simulink model "Assignment1_2"  (R2021a)
settings: Solver=VariableStepAuto  StartTime=0.0  StopTime=10.0  RelTol=1e-3
settings Model: Creator=mstra  LastModifiedBy=Luca
settings SolverCC: AlgebraicLoopSolver=TrustRegion
settings DebuggingCC: SFMachineParentedDataDiag=warning

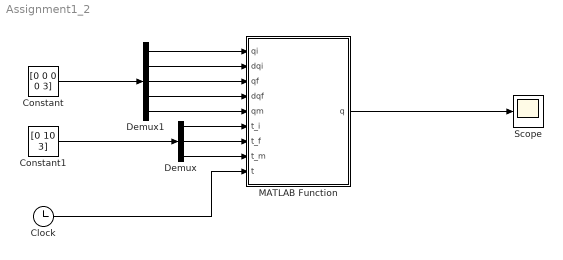
== system Assignment1_2 ==
  Clock : Clock
  Constant : Constant  Value=[0 0 0 0 3]
  Constant1 : Constant  Value=[0 10 3]
  Demux : Demux  Outputs=3
  Demux1 : Demux  Outputs=5
  MATLAB Function : MATLAB Function  TreatAsAtomicUnit=on
  Scope : Scope
  wires:
  Demux/1 -> MATLAB Function/6(t_i)
  Demux/2 -> MATLAB Function/7(t_f)
  Demux1/1 -> MATLAB Function/1(qi)
  Demux1/4 -> MATLAB Function/4(dqf)
  Constant1/1 -> Demux/1
  Constant/1 -> Demux1/1
  Clock/1 -> MATLAB Function/9(t)
  MATLAB Function/1(q) -> Scope/1
  Demux1/2 -> MATLAB Function/2(dqi)
  Demux1/3 -> MATLAB Function/3(qf)
  Demux1/5 -> MATLAB Function/5(qm)
  Demux/3 -> MATLAB Function/8(t_m)

== matlab function Assignment1_2/MATLAB Function ==
  data: qi input; dqi input; q output; qf input; dqf input; qm input; t_i input; t_f input; t_m input; t input
function q  = poly_trajD4(qi, dqi, qf, dqf, qm, t_i, t_f, t_m, t)
% poly_trajD4.m function returns the position at time t solving the 
% quartic polynomial. 
% INPUT:
% -	qi: initial value (i.e., value at t_i) 
% -	dqi: derivative at initial value (i.e., at time t_i) 
% -	qf: final value (i.e., value at time t_f) 
% -	dqf: derivative at final value (i.e., at time t_f) 
% -	qm: value at a generic intermediate time t_m, where t_i < t_m < t_f
% -	t_i: initial time 
% -	t_f: final time 
% -	t_m: generic intermediate time
% - t: symbolic time variable
% OUTPUT:
% - q: position at time t

% Construct the vector of variables and the matrix A 
v = [qi dqi qf dqf qm]';
A = [1   t_i    t_i^2    t_i^3      t_i^4;
     0   1      2*t_i    3*t_i^2    4*t_i^3;
     1   t_f    t_f^2    t_f^3      t_f^4;
     0   1      2*t_f    3*t_f^2    4*t_f^3;
     1   t_m    t_m^2    t_m^3      t_m^4   ];
% Solve the linear system to get the coefficients
a = A\v;
% Compute the position at time t with a quartic polynomial
q = a(1) + a(2).*(t-t_i) + a(3).*(t-t_i)^2 + a(4).*(t-t_i)^3 + a(5).*(t-t_i)^4;

end
